simulink model "pwm_control"  (Simulink 3.00)
libraries: mathlib x3, reglib x2, arclib x2, execlib x1

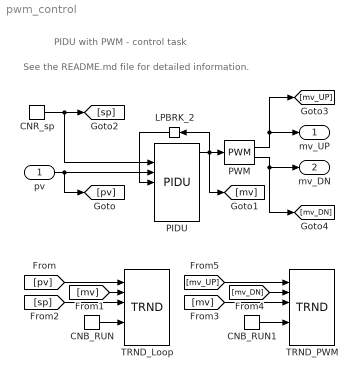
== system pwm_control ==
  note: See the README.md file for detailed information.
  note: PIDU with PWM - control task
  pv : Inport  Port=1
  CNB_RUN : mathlib/CNB  YCN=on
  CNB_RUN1 : mathlib/CNB  YCN=on
  CNR_sp : mathlib/CNR  ycn=0
  LPBRK_2 : execlib/LPBRK  Orientation=left
  PIDU : reglib/PIDU  irtype=7: PID  RACT=off  k=0.1  ti=10  td=2.5  nd=4  b=1  c=0  tt=1  hilim=1  lolim=-1  dz=0  icotype=1: Analog
  PWM : reglib/PWM  pertm=2  dtime=0.1  btime=0.1  offtime=0.1  asyfac=1  SYNCH=off
  TRND_Loop : arclib/TRND  n=3  l=100  btype=8  ptype1=1: Store  ptype2=1: Store  ptype3=1: Store  ptype4=1: Store  pfac=1  afac=0  arc=0  id=1  Title=Trend Title  timesrc=1
  TRND_PWM : arclib/TRND  n=3  l=100  btype=8  ptype1=1: Store  ptype2=1: Store  ptype3=1: Store  ptype4=1: Store  pfac=1  afac=0  arc=0  id=2  Title=Trend Title  timesrc=1
  mv_UP : Outport  Port=1
  mv_DN : Outport  Port=2
  wires:
  CNB_RUN/1 -> TRND_Loop/5
  CNB_RUN1/1 -> TRND_PWM/5
  CNR_sp/1 -> [sp], PIDU/2
  [pv] -> TRND_Loop/1
  [mv] -> TRND_Loop/2
  [sp] -> TRND_Loop/3
  [mv] -> TRND_PWM/3
  [mv_DN] -> TRND_PWM/2
  [mv_UP] -> TRND_PWM/1
  LPBRK_2/1 -> PIDU/4
  PIDU/1 -> [mv], LPBRK_2/1, PWM/1
  PWM/1 -> [mv_UP], mv_UP/1
  PWM/2 -> [mv_DN], mv_DN/1
  pv/1 -> [pv], PIDU/3
